simulink model "lab4_1"  (R2022a)
settings: Solver=VariableStepAuto  StartTime=0.0  StopTime=Tmdl  FixedStep=To/100  MaxStep=To/100  RelTol=1e-3
undefined symbols (not defined in the file or in its folder): an, dsc, k, To
settings Model: Creator=Professional  LastModifiedBy=osini

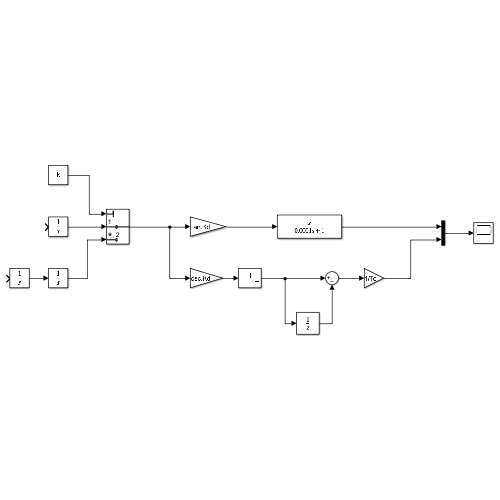
[thumbnail: Simulink's stored preview of the top-level diagram]
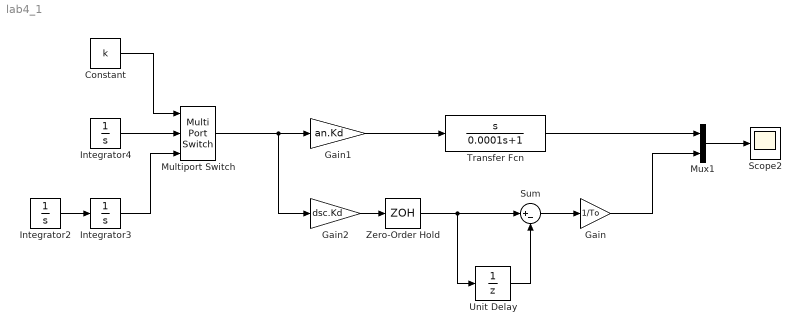
== system lab4_1 ==
  Constant : Constant  Value=k
  Gain : Gain  Gain=1/To
  Gain1 : Gain  Gain=an.Kd
  Gain2 : Gain  Gain=dsc.Kd
  Integrator2 : Integrator  InitialCondition=1
  Integrator3 : Integrator
  Integrator4 : Integrator  InitialCondition=1
  Multiport Switch : MultiPortSwitch  Inputs=2  SaturateOnIntegerOverflow=off  InputSameDT=off
  Mux1 : Mux  Inputs=2
  Scope2 : Scope
  Sum : Sum  Inputs=|+-
  Transfer Fcn : TransferFcn  Numerator=[1 0]  Denominator=[0.0001 1]
  Unit Delay : UnitDelay  SampleTime=-1  HasFrameUpgradeWarning=on
  Zero-Order Hold : ZeroOrderHold  SampleTime=To
  wires:
  Mux1/1 -> Scope2/1
  Gain2/1 -> Zero-Order Hold/1
  Gain1/1 -> Transfer Fcn/1
  Multiport Switch/1 -> Gain2/1, Gain1/1
  Zero-Order Hold/1 -> Unit Delay/1, Sum/1
  Sum/1 -> Gain/1
  Transfer Fcn/1 -> Mux1/1
  Gain/1 -> Mux1/2
  Unit Delay/1 -> Sum/2
  Integrator2/1 -> Integrator3/1
  Integrator4/1 -> Multiport Switch/2
  Constant/1 -> Multiport Switch/1
  Integrator3/1 -> Multiport Switch/3
